simulink model "state_estimator_opt_driftingcar"  (R2017a)
settings: Solver=FixedStepAuto  StartTime=0.0  StopTime=inf  FixedStep=1/150  RelTol=1e-3
InitFcn:
  | state_estimator_opt_driftingcar_callback
values from neighbouring files (symbols this model uses):
  ds_nonzero_threshold = 1e-3    (= 0.001)    [state_estimator_opt_driftingcar_callback.m]
undefined symbols (not defined in the file or in its folder): magnitude
libraries: robotlib x7, simulink x5, dspsigops x2, sharedtransform x1
settings Model: Creator=marco  LastModifiedBy=marco
settings OptimizationCC: PassReuseOutputArgsAs=Individual arguments  MaxStackSize=64
settings DebuggingCC: ParameterTunabilityLossMsg=error
settings HardwareCC: ProdBitPerPointer=32  ProdBitPerSizeT=32  ProdBitPerPtrDiffT=32  ProdLargestAtomicFloat=None  ProdIntDivRoundTo=Undefined  ProdEndianess=Unspecified  ProdWordSize=32  ProdHWDeviceType=Generic->Unspecified (assume 32-bit Generic)
settings SFSimCC: MATLABDynamicMemAlloc=off
settings RTWCC: SystemTargetFile=ert.tlc  HardwareBoard=Robot Operating System (ROS)  TLCOptions="-aInlineSetEventsForThisBaseRateFcn=TLC_FALSE -aSuppressMultiTaskScheduler=TLC_FALSE  -aRateBasedStepFcn=0"  TemplateMakefile=ert_default_tmf  Description=Embedded Coder  GenerateReport=on  Toolchain=Catkin  IncludeHyperlinkInReport=on  LaunchReport=on  TargetLang=C++  GenerateTraceInfo=on  GenerateTraceReport=on  GenerateTraceReportSl=on  GenerateTraceReportSf=on  GenerateTraceReportEml=on
settings CodeAppCC: ForceParamTrailComments=on  IgnoreCustomStorageClasses=off  OperatorAnnotations=on  SimulinkDataObjDesc=on  SFDataObjDesc=on  MATLABFcnDesc=on  InsertBlockDesc=on  MATLABSourceComments=on

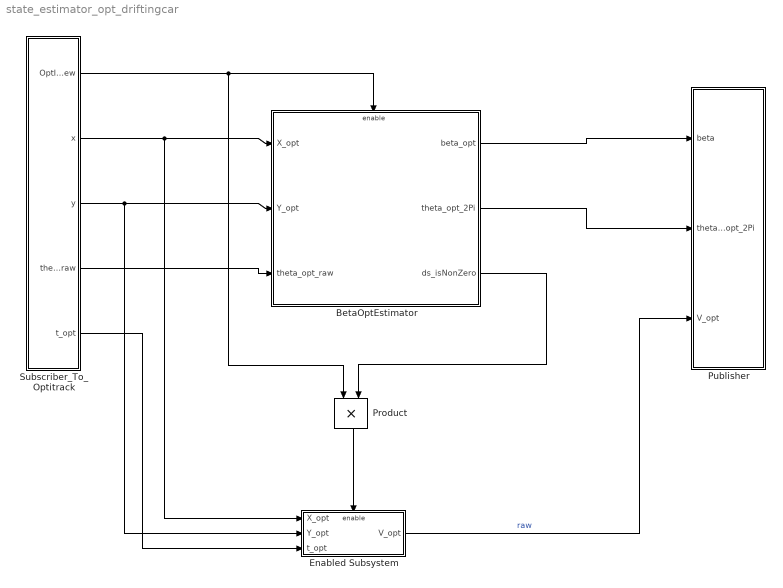
== system state_estimator_opt_driftingcar ==
  BetaOptEstimator : Subsystem
  Enabled Subsystem : Subsystem  TreatAsAtomicUnit=on
  Product : Product
  Publisher : Subsystem
  Subscriber_To_Optitrack : Subsystem
  wires:
  Subscriber_To_Optitrack/1(OptIsNew) -> Product/1, BetaOptEstimator/Enable
  Subscriber_To_Optitrack/4(theta_opt_raw) -> BetaOptEstimator/3(theta_opt_raw)
  BetaOptEstimator/1(beta_opt) -> Publisher/1(beta)
  BetaOptEstimator/2(theta_opt_2Pi) -> Publisher/2(theta_opt_2Pi)
  Subscriber_To_Optitrack/5(t_opt) -> Enabled Subsystem/3(t_opt)
  Enabled Subsystem/1(V_opt) -> Publisher/3(V_opt)  "raw"
  Product/1 -> Enabled Subsystem/Enable
  Subscriber_To_Optitrack/2(x) -> Enabled Subsystem/1(X_opt), BetaOptEstimator/1(X_opt)
  Subscriber_To_Optitrack/3(y) -> Enabled Subsystem/2(Y_opt), BetaOptEstimator/2(Y_opt)
  BetaOptEstimator/3(ds_isNonZero) -> Product/2

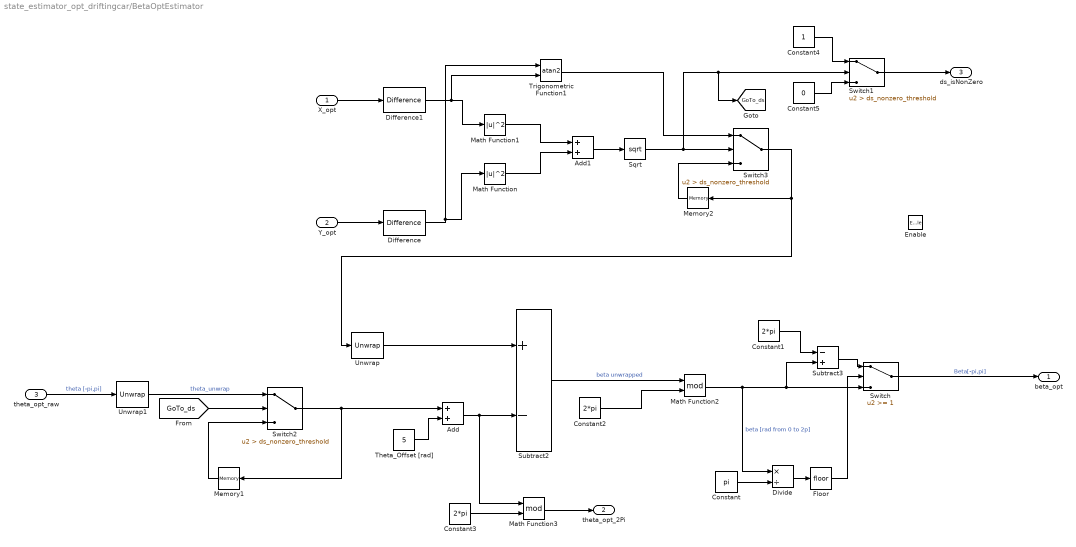
== system state_estimator_opt_driftingcar/BetaOptEstimator ==
  X_opt : Inport
  Y_opt : Inport  Port=2
  theta_opt_raw : Inport  Port=3
  Enable : EnablePort
  Add : Sum
  Add1 : Sum
  Constant : Constant  Value=pi
  Constant1 : Constant  Value=2*pi
  Constant2 : Constant  Value=2*pi
  Constant3 : Constant  Value=2*pi
  Constant4 : Constant
  Constant5 : Constant  Value=0
  Difference : simulink/Discrete/Difference  ICPrevInput=0.0  OutMin=[]  OutMax=[]  OutDataType=fixdt(1, 16)  OutScaling=2^-10  DoSatur=off
  Difference1 : simulink/Discrete/Difference  ICPrevInput=0.0  OutMin=[]  OutMax=[]  OutDataType=fixdt(1, 16)  OutScaling=2^-10  DoSatur=off
  Divide : Product  Inputs=*/
  Floor : Rounding
  Math Function : Math  Operator=magnitude^2  SaturateOnIntegerOverflow=on
  Math Function1 : Math  Operator=magnitude^2  SaturateOnIntegerOverflow=on
  Math Function2 : Math  Operator=mod  SaturateOnIntegerOverflow=on
  Math Function3 : Math  Operator=mod  SaturateOnIntegerOverflow=on
  Memory1 : Memory
  Memory2 : Memory
  Sqrt : Sqrt  SaturateOnIntegerOverflow=on
  Subtract2 : Sum  Inputs=+-
  Subtract3 : Sum  Inputs=-+
  Switch : Switch  Threshold=1
  Switch1 : Switch  Criteria=u2 > Threshold  Threshold=ds_nonzero_threshold
  Switch2 : Switch  Criteria=u2 > Threshold  Threshold=ds_nonzero_threshold
  Switch3 : Switch  Criteria=u2 > Threshold  Threshold=ds_nonzero_threshold
  Theta_Offset [rad] : Constant  Value=5
  Trigonometric Function1 : Trigonometry  Operator=atan2
  Unwrap : dspsigops/Unwrap  tol=pi  InputProcessing=Columns as channels (frame based)  running=off
  Unwrap1 : dspsigops/Unwrap  tol=pi  InputProcessing=Columns as channels (frame based)  running=off
  beta_opt : Outport
  theta_opt_2Pi : Outport  Port=2
  ds_isNonZero : Outport  Port=3
  tag scope: GoTo_ds=global
  wires:
  X_opt/1 -> Difference1/1
  Constant/1 -> Divide/2
  Divide/1 -> Floor/1
  Constant2/1 -> Math Function2/2
  Subtract3/1 -> Switch/1
  Subtract2/1 -> Math Function2/1  "beta unwrapped"
  Unwrap/1 -> Subtract2/1
  Math Function2/1 -> Divide/1, Subtract3/2, Switch/3  "beta [rad from 0 to 2p]"
  Floor/1 -> Switch/2
  Switch/1 -> beta_opt/1  "Beta[-pi,pi]"
  theta_opt_raw/1 -> Unwrap1/1  "theta [-pi,pi]"
  Theta_Offset [rad]/1 -> Add/2
  Add/1 -> Math Function3/1, Subtract2/2
  Constant1/1 -> Subtract3/1
  Y_opt/1 -> Difference/1
  Math Function1/1 -> Add1/1
  Difference/1 -> Trigonometric Function1/1, Math Function/1
  Switch3/1 -> Unwrap/1, Memory2/1
  Difference1/1 -> Trigonometric Function1/2, Math Function1/1
  Add1/1 -> Sqrt/1
  Math Function/1 -> Add1/2
  Sqrt/1 -> [GoTo_ds], Switch1/2, Switch3/2
  Memory2/1 -> Switch3/3
  Trigonometric Function1/1 -> Switch3/1
  Constant3/1 -> Math Function3/2
  Math Function3/1 -> theta_opt_2Pi/1
  Constant5/1 -> Switch1/3
  Constant4/1 -> Switch1/1
  Switch1/1 -> ds_isNonZero/1
  Memory1/1 -> Switch2/3
  Unwrap1/1 -> Switch2/1  "theta_unwrap"
  Switch2/1 -> Memory1/1, Add/1
  [GoTo_ds] -> Switch2/2

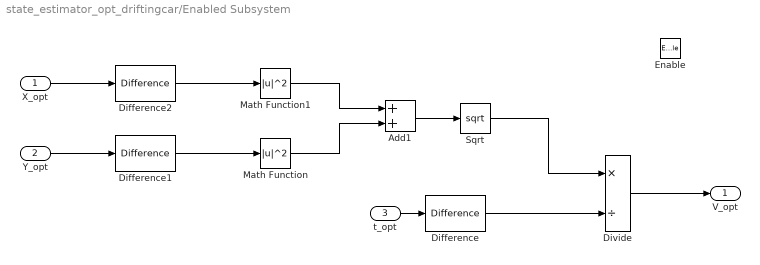
== system state_estimator_opt_driftingcar/Enabled Subsystem ==
  X_opt : Inport
  Y_opt : Inport  Port=2
  t_opt : Inport  Port=3
  Enable : EnablePort
  Add1 : Sum
  Difference : simulink/Discrete/Difference  ICPrevInput=0.0  OutMin=[]  OutMax=[]  OutDataType=fixdt(1, 16)  OutScaling=2^-10  DoSatur=off
  Difference1 : simulink/Discrete/Difference  ICPrevInput=0.0  OutMin=[]  OutMax=[]  OutDataType=fixdt(1, 16)  OutScaling=2^-10  DoSatur=off
  Difference2 : simulink/Discrete/Difference  ICPrevInput=0.0  OutMin=[]  OutMax=[]  OutDataType=fixdt(1, 16)  OutScaling=2^-10  DoSatur=off
  Divide : Product  Inputs=*/
  Math Function : Math  Operator=magnitude^2  SaturateOnIntegerOverflow=on
  Math Function1 : Math  Operator=magnitude^2  SaturateOnIntegerOverflow=on
  Sqrt : Sqrt  SaturateOnIntegerOverflow=on
  V_opt : Outport
  wires:
  t_opt/1 -> Difference/1
  Divide/1 -> V_opt/1
  Difference/1 -> Divide/2
  Difference2/1 -> Math Function1/1
  Math Function/1 -> Add1/2
  Difference1/1 -> Math Function/1
  Sqrt/1 -> Divide/1
  Y_opt/1 -> Difference1/1
  Math Function1/1 -> Add1/1
  Add1/1 -> Sqrt/1
  X_opt/1 -> Difference2/1

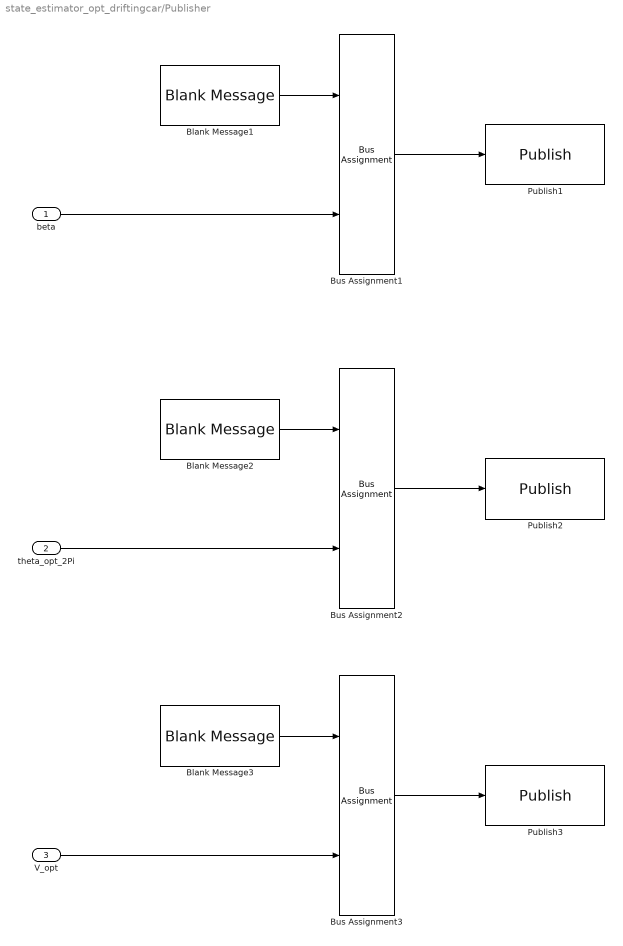
== system state_estimator_opt_driftingcar/Publisher ==
  beta : Inport
  theta_opt_2Pi : Inport  Port=2
  V_opt : Inport  Port=3
  Blank Message1 : robotlib/Blank Message  SourceLibraryInfo=This block requires Robotics System Toolbox  messageType=std_msgs/Float64  SampleTime=inf
      settings: SourceProductBaseCode=RO
  Blank Message2 : robotlib/Blank Message  SourceLibraryInfo=This block requires Robotics System Toolbox  messageType=std_msgs/Float64  SampleTime=inf
      settings: SourceProductBaseCode=RO
  Blank Message3 : robotlib/Blank Message  SourceLibraryInfo=This block requires Robotics System Toolbox  messageType=std_msgs/Float64  SampleTime=inf
      settings: SourceProductBaseCode=RO
  Bus Assignment1 : BusAssignment  AssignedSignals=Data
  Bus Assignment2 : BusAssignment  AssignedSignals=Data
  Bus Assignment3 : BusAssignment  AssignedSignals=Data
  Publish1 : robotlib/Publish  SourceLibraryInfo=This block requires Robotics System Toolbox  topicSource=Specify your own  topic=/state_estimator_opt_beta  messageType=std_msgs/Float64  messageQueueLength=1
      settings: SourceProductBaseCode=RO
  Publish2 : robotlib/Publish  SourceLibraryInfo=This block requires Robotics System Toolbox  topicSource=Specify your own  topic=/state_estimator_opt_theta  messageType=std_msgs/Float64  messageQueueLength=1
      settings: SourceProductBaseCode=RO
  Publish3 : robotlib/Publish  SourceLibraryInfo=This block requires Robotics System Toolbox  topicSource=Specify your own  topic=/state_estimator_opt_V  messageType=std_msgs/Float64  messageQueueLength=1
      settings: SourceProductBaseCode=RO
  wires:
  beta/1 -> Bus Assignment1/2
  Blank Message1/1 -> Bus Assignment1/1
  Bus Assignment1/1 -> Publish1/1
  theta_opt_2Pi/1 -> Bus Assignment2/2
  Blank Message2/1 -> Bus Assignment2/1
  Bus Assignment2/1 -> Publish2/1
  V_opt/1 -> Bus Assignment3/2
  Blank Message3/1 -> Bus Assignment3/1
  Bus Assignment3/1 -> Publish3/1

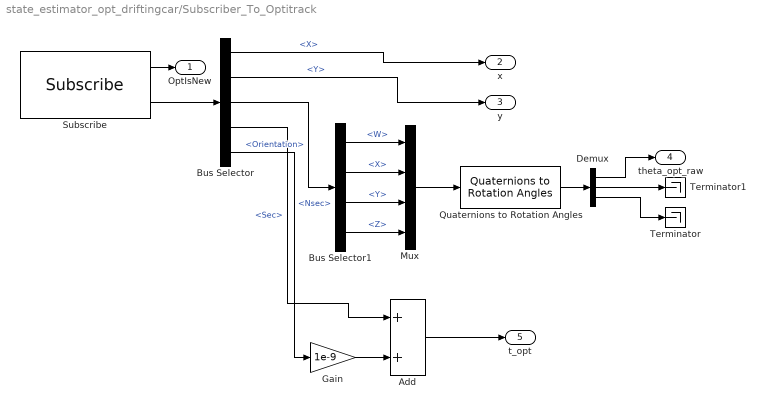
== system state_estimator_opt_driftingcar/Subscriber_To_Optitrack ==
  Add : Sum
  Bus Selector : BusSelector  OutputSignals=Pose.Position.X,Pose.Position.Y,Pose.Orientation,Header.Stamp.Sec,Header.Stamp.Nsec
  Bus Selector1 : BusSelector  OutputSignals=W,X,Y,Z
  Demux : Demux  Outputs=3
  Gain : Gain  Gain=1e-9
  Mux : Mux
  Quaternions to Rotation Angles : sharedtransform/Quaternions to Rotation Angles  rotationOrder=ZYX
  Subscribe : robotlib/Subscribe  SourceLibraryInfo=This block requires Robotics System Toolbox  topicSource=Specify your own  topic=/car/pose  messageType=geometry_msgs/PoseStamped  sampleTime=-1  messageQueueLength=1
      settings: SourceProductBaseCode=RO
  Terminator : Terminator
  Terminator1 : Terminator
  OptIsNew : Outport
  x : Outport  Port=2
  y : Outport  Port=3
  theta_opt_raw : Outport  Port=4
  t_opt : Outport  Port=5
  wires:
  Subscribe/2 -> Bus Selector/1
  Subscribe/1 -> OptIsNew/1
  Bus Selector/1 -> x/1  "<X>"
  Bus Selector/2 -> y/1  "<Y>"
  Quaternions to Rotation Angles/1 -> Demux/1
  Demux/3 -> Terminator/1
  Demux/2 -> Terminator1/1
  Demux/1 -> theta_opt_raw/1
  Mux/1 -> Quaternions to Rotation Angles/1
  Bus Selector/3 -> Bus Selector1/1  "<Orientation>"
  Bus Selector1/1 -> Mux/1  "<W>"
  Bus Selector1/2 -> Mux/2  "<X>"
  Bus Selector1/3 -> Mux/3  "<Y>"
  Bus Selector1/4 -> Mux/4  "<Z>"
  Gain/1 -> Add/2
  Bus Selector/5 -> Gain/1  "<Nsec>"
  Bus Selector/4 -> Add/1  "<Sec>"
  Add/1 -> t_opt/1
